simulink model "test_eb_astitsmc_comp_formation_xy_gazebo_final"  (R2023a)
settings: Solver=FixedStepAuto  StartTime=0.0  StopTime=inf  FixedStep=0.07  RelTol=1e-3
undefined symbols (not defined in the file): angular, DiscIntNeverNeededParam, linear
libraries: ros2lib x14, simulink x4, robotcorelib x4
(part 2 of 2)

== matlab function test_eb_astitsmc_comp_formation_xy_gazebo_final/Translational Control3/Flocking1/MATLAB Function ==
  data: xi input; yi input; phiAlpha output; xj input; yj input; xk input; yk input; xl input; yl input; params input

function phiAlpha  = phiAlphaFcn(xi, yi, xj, yj, xk, yk, xl, yl, params)
    
    % Flocking parameters
    epsilon = params(1); a = params(2); b = params(3); c = params(4); d = params(5); h = params(6);

    e = abs(a - b) / sqrt(4*a*b) ;

    cAlpha = sigmaNormFun(c, epsilon) ;
    dAlpha = sigmaNormFun(d, epsilon) ;

    %%
    Pi = [xi;yi] ;
    Pj = [xj;yj] ;
    Pk = [xk;yk] ;
    Pl = [xl;yl] ;

    %%
    sigmaNormj = sigmaNormFun(Pj - Pi, epsilon) ;
    nij = gradSigmaFun(Pj - Pi, epsilon) ;
    
    sigmaNormk = sigmaNormFun(Pk - Pi, epsilon) ;
    nik = gradSigmaFun(Pk - Pi, epsilon) ;

    sigmaNorml = sigmaNormFun(Pl - Pi, epsilon) ;
    nil = gradSigmaFun(Pl - Pi, epsilon) ;

    %%
    sigma1j = sigma1Fun(sigmaNormj - dAlpha + e) ;
    sigma1k = sigma1Fun(sigmaNormk - dAlpha + e) ;
    sigma1l = sigma1Fun(sigmaNorml - dAlpha + e) ;
            
    %% Position
    phiAlphaj = 0.5 * bumpFcn(sigmaNormj/cAlpha,h) * ((a+b)*sigma1j + (a-b)) ;
    phiAlphanij = phiAlphaj.* nij ;
    
    phiAlphak = 0.5 * bumpFcn(sigmaNormk/cAlpha,h) * ((a+b)*sigma1k + (a-b)) ;
    phiAlphanik = phiAlphak.* nik ;

    phiAlphal = 0.5 * bumpFcn(sigmaNorml/cAlpha,h) * ((a+b)*sigma1l + (a-b)) ;
    phiAlphanil = phiAlphal.* nil ;

    phiAlpha = phiAlphanij + phiAlphanik + phiAlphanil;

    
end

== matlab function test_eb_astitsmc_comp_formation_xy_gazebo_final/Translational Control3/Flocking1/MATLAB Function1 ==
  data: phiAlpha input; phiAlpha_int input; ui_gamma input; yaw input; Ui_pos output size=3; ui_yaw output; KP input; eyaw output size=1; eyaw1 input; eyaw2 input; eyaw4 input

function [Ui_pos, ui_yaw, eyaw]  = ctrlLaw(phiAlpha, phiAlpha_int, ui_gamma, yaw, KP, eyaw1, eyaw2, eyaw4)  %, phiBetak, bikobs, phiBetanei, bikve
    
    % Control gains and parameters
    Kx = KP(1); Ky = KP(2); Kz = KP(3);
    Kix = KP(4); Kiy = KP(5); Kiz = KP(6);
    Kyaw = KP(7); Kdyaw = KP(8);
    off = KP(9);

    eyaw = 0 - yaw(1);
    deyaw = 0 - yaw(2);


    ui_yaw = Kyaw*eyaw + Kdyaw*deyaw;
    hz_dot = ui_gamma(3,1);  %+ cBetaz * (phiBetak(3,1) + phiBetanei(3,1)) + cdBetaz * (bikobs(3,1) + bikve(3,1));

    if eyaw < off && eyaw > -off % && eyaw1 < off && eyaw1 > -off && eyaw2 < off && eyaw2 > -off && eyaw4 < off && eyaw4 > -off
        hx_dot = Kx * phiAlpha(1,1) + Kix * phiAlpha_int(1,1) + ui_gamma(1,1);  %+ cBetax * (phiBetak(1,1) + phiBetanei(1,1)) + cdBetax * (bikobs(1,1) + bikve(1,1));
        hy_dot = Ky * phiAlpha(2,1) + Kiy * phiAlpha_int(2,1) + ui_gamma(2,1);  %+ cBetay * (phiBetak(2,1) + phiBetanei(2,1)) + cdBetay * (bikobs(2,1) + bikve(2,1));
    else
        hx_dot = 0;
        hy_dot = 0;
    end
    

    Ui_pos = [hx_dot; hy_dot; hz_dot] ;
    

end

== matlab function test_eb_astitsmc_comp_formation_xy_gazebo_final/Translational Control3/Flocking1/MATLAB Function2 ==
  data: ui_prev input; xi input; yi input; zi input; ui_gamma output size=3; xr input; yr input; zr input; xr2 input; yr2 input; zr2 input; fig input; err output size=3; K_cts input; K_sw input; norm_Vex input; norm_Vey input; norm_Vez input; i_terminal input size=3; ETA input size=3; V2 input size=3; terminal output size=3; dot_ETA output size=3; dot_V2 output
function [ui_gamma, err, terminal, dot_ETA, dot_V2] = naviFeedback(ui_prev, xi, yi, zi, xr, yr, zr, xr2, yr2, zr2, fig, K_cts, K_sw, norm_Vex, norm_Vey, norm_Vez, i_terminal, ETA, V2)
    
    Kp = K_cts(1); Kpz = K_cts(2); C = K_cts(3); Cz = K_cts(4); alphaxy = K_cts(5); alphaz = K_cts(6);
    gammaxy = K_sw(1); gammaz = K_sw(2); alpha1xy = K_sw(3); alpha1z = K_sw(4); alpha2xy = K_sw(5); alpha2z = K_sw(6);

    %Sepration control
    ui_xprev = ui_prev(1); ui_yprev = ui_prev(2); ui_zprev = ui_prev(3);
    
    if fig == 1
        e_x = (xr - xi - 0.5) + (xr2 - xi - 1);
        e_y = (yr - yi - 0.5) + (yr2 - yi);
        e_z = (zr - zi + 0.1) + (zr2 - zi);
    elseif fig == 2
        e_x = (xr - xi + 0.5) + (xr2 - xi);
        e_y = (yr - yi - 0.5) + (yr2 - yi - 1);
        e_z = (zr - zi - 0.1) + (zr2 - zi);
    else
        e_x = (xr - xi + 0.5) + (xr2 - xi);
        e_y = (yr - yi - 0.5) + (yr2 - yi - 1);
        e_z = (zr - zi - 0.5) + (zr2 - zi - 0.6);
    end

    err = [e_x;e_y;e_z];

    term_1 = abs(e_x)^(alphaxy)*sign(e_x);
    term_2 = abs(e_y)^(alphaxy)*sign(e_y);
    term_3 = abs(e_z)^(alphaz)*sign(e_z);

    terminal = [term_1;term_2;term_3];

    %Manifold definitions
    Sx = e_x + C*i_terminal(1);
    Sy = e_y + C*i_terminal(2);
    Sz = e_z + Cz*i_terminal(3);

    %Disturbance estimate adaptation
    dot_eta_x = gammaxy*abs(Sx) - 0.001*ETA(1);
    dot_eta_y = gammaxy*abs(Sy) - 0.001*ETA(2);
    dot_eta_z = gammaz*abs(Sz) - 0.001*ETA(3);
    dot_ETA = [dot_eta_x;dot_eta_y;dot_eta_z];

    k1x = alpha1xy*sqrt(ETA(1));
    k1y = alpha1xy*sqrt(ETA(2));
    k1z = alpha1z*sqrt(ETA(3));

    k2x = alpha2xy*ETA(1);
    k2y = alpha2xy*ETA(2);
    k2z = alpha2z*ETA(3);

    %Switching law
    v1x = ETA(1)*tanh(Sx);
    v1y = ETA(2)*tanh(Sy);
    v1z = ETA(3)*tanh(Sz);
    
    dot_v2x = 0.001*tanh(Sx);
    dot_v2y = 0.001*tanh(Sy);
    dot_v2z = 0.0015*tanh(Sz);
    dot_V2 = [dot_v2x;dot_v2y;dot_v2z];

    % ux = 0 + v1x;
    % uy = 0 + v1y;
    % uz = 0 + v1z;

    %Final control law
    if  norm_Vex >= 0
        ux = 0 + v1x;
    else
        ux = ui_xprev;
    end

    if  norm_Vey >= 0
        uy = 0 + v1y;
    else
        uy = ui_yprev;
    end

    if  norm_Vez >= 0
        uz = 0 + v1z;
    else
        uz = ui_zprev;
    end

    ui_gamma = [ux;uy;uz];
    
end

== matlab function test_eb_astitsmc_comp_formation_xy_gazebo_final/Translational Control4/event_2 ==
  data: e_t output; X_d input; X_d2 input; X input; Kevs input; fig input
function e_t  = fcn(X_d, X_d2, X, Kevs, fig)

%Separation of desired and actual positions, velocities ans accelerations in their components
X_l = X_d(1:6); 
xr = X_l(1);    vxr = X_l(4);      
yr = X_l(2);    vyr = X_l(5);   
zr = X_l(3);    vzr = X_l(6);   

X_l2 = X_d2(1:4); 
xr2 = X_l2(1);    
yr2 = X_l2(2);    
zr2 = X_l2(3);    

X_a = X(1:3);
xi = X_a(1);     
yi = X_a(2);     
zi = X_a(3);     

%Parameters separation ans designation
c0x = Kevs(1);
c0y = Kevs(2);
c0z = Kevs(3);

%Errors definition (position and velocity)
if fig == 1
        ex = (xr - xi + 0.5) + (xr2 - xi);
        ey = (yr - yi - 0.5) + (yr2 - yi - 1);
        ez = (zr - zi - 0.1) + (zr2 - zi);
elseif fig == 2
        ex = (xr - xi + 0.5) + (xr2 - xi + 1);
        ey = (yr - yi + 0.5) + (yr2 - yi);
        ez = (zr - zi + 0.1) + (zr2 - zi);
else
        ex = (xr - xi + 0.5) + (xr2 - xi + 1);
        ey = (yr - yi + 0.5) + (yr2 - yi);
        ez = (zr - zi + 0.1) + (zr2 - zi);
end

e_x = abs(ex) - c0x;
e_y = abs(ey) - c0y;
e_z = abs(ez) - c0z;

e_t = [e_x;e_y;e_z];

== matlab function test_eb_astitsmc_comp_formation_xy_gazebo_final/Translational Control4/Flocking1/MATLAB Function ==
  data: xi input; yi input; phiAlpha output; xj input; yj input; xk input; yk input; xl input; yl input; params input

function phiAlpha  = phiAlphaFcn(xi, yi, xj, yj, xk, yk, xl, yl, params)
    
    % Flocking parameters
    epsilon = params(1); a = params(2); b = params(3); c = params(4); d = params(5); h = params(6);

    e = abs(a - b) / sqrt(4*a*b) ;

    cAlpha = sigmaNormFun(c, epsilon) ;
    dAlpha = sigmaNormFun(d, epsilon) ;

    %%
    Pi = [xi;yi] ;
    Pj = [xj;yj] ;
    Pk = [xk;yk] ;
    Pl = [xl;yl] ;

    %%
    sigmaNormj = sigmaNormFun(Pj - Pi, epsilon) ;
    nij = gradSigmaFun(Pj - Pi, epsilon) ;
    
    sigmaNormk = sigmaNormFun(Pk - Pi, epsilon) ;
    nik = gradSigmaFun(Pk - Pi, epsilon) ;

    sigmaNorml = sigmaNormFun(Pl - Pi, epsilon) ;
    nil = gradSigmaFun(Pl - Pi, epsilon) ;

    %%
    sigma1j = sigma1Fun(sigmaNormj - dAlpha + e) ;
    sigma1k = sigma1Fun(sigmaNormk - dAlpha + e) ;
    sigma1l = sigma1Fun(sigmaNorml - dAlpha + e) ;
            
    %% Position
    phiAlphaj = 0.5 * bumpFcn(sigmaNormj/cAlpha,h) * ((a+b)*sigma1j + (a-b)) ;
    phiAlphanij = phiAlphaj.* nij ;
    
    phiAlphak = 0.5 * bumpFcn(sigmaNormk/cAlpha,h) * ((a+b)*sigma1k + (a-b)) ;
    phiAlphanik = phiAlphak.* nik ;

    phiAlphal = 0.5 * bumpFcn(sigmaNorml/cAlpha,h) * ((a+b)*sigma1l + (a-b)) ;
    phiAlphanil = phiAlphal.* nil ;

    phiAlpha = phiAlphanij + phiAlphanik + phiAlphanil;

    
end

== matlab function test_eb_astitsmc_comp_formation_xy_gazebo_final/Translational Control4/Flocking1/MATLAB Function1 ==
  data: phiAlpha input; phiAlpha_int input; ui_gamma input; yaw input; Ui_pos output size=3; ui_yaw output; KP input; eyaw output size=1; eyaw1 input; eyaw2 input; eyaw3 input

function [Ui_pos, ui_yaw, eyaw]  = ctrlLaw(phiAlpha, phiAlpha_int, ui_gamma, yaw, KP, eyaw1, eyaw2, eyaw3)  %, phiBetak, bikobs, phiBetanei, bikve
    
    % Control gains and parameters
    Kx = KP(1); Ky = KP(2); Kz = KP(3);
    Kix = KP(4); Kiy = KP(5); Kiz = KP(6);
    Kyaw = KP(7); Kdyaw = KP(8);
    off = KP(9);

    eyaw = 0 - yaw(1);
    deyaw = 0 - yaw(2);


    ui_yaw = Kyaw*eyaw + Kdyaw*deyaw;
    hz_dot = ui_gamma(3,1);  %+ cBetaz * (phiBetak(3,1) + phiBetanei(3,1)) + cdBetaz * (bikobs(3,1) + bikve(3,1));

    if eyaw < off && eyaw > -off % && eyaw1 < off && eyaw1 > -off && eyaw2 < off && eyaw2 > -off && eyaw3 < off && eyaw3 > -off
        hx_dot = Kx * phiAlpha(1,1) + Kix * phiAlpha_int(1,1) + ui_gamma(1,1);  %+ cBetax * (phiBetak(1,1) + phiBetanei(1,1)) + cdBetax * (bikobs(1,1) + bikve(1,1));
        hy_dot = Ky * phiAlpha(2,1) + Kiy * phiAlpha_int(2,1) + ui_gamma(2,1);  %+ cBetay * (phiBetak(2,1) + phiBetanei(2,1)) + cdBetay * (bikobs(2,1) + bikve(2,1));
    else
        hx_dot = 0;
        hy_dot = 0;
    end
    

    Ui_pos = [hx_dot; hy_dot; hz_dot] ;
    

end

== matlab function test_eb_astitsmc_comp_formation_xy_gazebo_final/Translational Control1/Flocking1/MATLAB Function ==
  data: xi input; yi input; phiAlpha output; xj input; yj input; xk input; yk input; xl input; yl input; params input

function phiAlpha  = phiAlphaFcn(xi, yi, xj, yj, xk, yk, xl, yl, params)
    
    % Flocking parameters
    epsilon = params(1); a = params(2); b = params(3); c = params(4); d = params(5); h = params(6);

    e = abs(a - b) / sqrt(4*a*b) ;

    cAlpha = sigmaNormFun(c, epsilon) ;
    dAlpha = sigmaNormFun(d, epsilon) ;

    %%
    Pi = [xi;yi] ;
    Pj = [xj;yj] ;
    Pk = [xk;yk] ;
    Pl = [xl;yl] ;

    %%
    sigmaNormj = sigmaNormFun(Pj - Pi, epsilon) ;
    nij = gradSigmaFun(Pj - Pi, epsilon) ;
    
    sigmaNormk = sigmaNormFun(Pk - Pi, epsilon) ;
    nik = gradSigmaFun(Pk - Pi, epsilon) ;

    sigmaNorml = sigmaNormFun(Pl - Pi, epsilon) ;
    nil = gradSigmaFun(Pl - Pi, epsilon) ;

    %%
    sigma1j = sigma1Fun(sigmaNormj - dAlpha + e) ;
    sigma1k = sigma1Fun(sigmaNormk - dAlpha + e) ;
    sigma1l = sigma1Fun(sigmaNorml - dAlpha + e) ;
            
    %% Position
    phiAlphaj = 0.5 * bumpFcn(sigmaNormj/cAlpha,h) * ((a+b)*sigma1j + (a-b)) ;
    phiAlphanij = phiAlphaj.* nij ;
    
    phiAlphak = 0.5 * bumpFcn(sigmaNormk/cAlpha,h) * ((a+b)*sigma1k + (a-b)) ;
    phiAlphanik = phiAlphak.* nik ;

    phiAlphal = 0.5 * bumpFcn(sigmaNorml/cAlpha,h) * ((a+b)*sigma1l + (a-b)) ;
    phiAlphanil = phiAlphal.* nil ;

    phiAlpha = phiAlphanij + phiAlphanik + phiAlphanil;

    
end

== matlab function test_eb_astitsmc_comp_formation_xy_gazebo_final/Translational Control1/Flocking1/MATLAB Function1 ==
  data: phiAlpha input; phiAlpha_int input; ui_gamma input; yaw input; Ui_pos output size=3; ui_yaw output; KP input; eyaw output size=1; eyaw2 input; eyaw3 input; eyaw4 input

function [Ui_pos, ui_yaw, eyaw]  = ctrlLaw(phiAlpha, phiAlpha_int, ui_gamma, yaw, KP, eyaw2, eyaw3, eyaw4)  %, phiBetak, bikobs, phiBetanei, bikve
    
    % Control gains and parameters
    Kx = KP(1); Ky = KP(2); Kz = KP(3);
    Kix = KP(4); Kiy = KP(5); Kiz = KP(6);
    Kyaw = KP(7); Kdyaw = KP(8);
    off = KP(9);


    eyaw = 0 - yaw(1);
    deyaw = 0 - yaw(2);


    ui_yaw = Kyaw*eyaw + Kdyaw*deyaw;
    hz_dot = ui_gamma(3,1);  %+ cBetaz * (phiBetak(3,1) + phiBetanei(3,1)) + cdBetaz * (bikobs(3,1) + bikve(3,1));

    if eyaw < off && eyaw > -off % && eyaw2 < off && eyaw2 > -off  && eyaw3 < off && eyaw3 > -off && eyaw4 < off && eyaw4 > -off
        hx_dot = Kx * phiAlpha(1,1) + Kix * phiAlpha_int(1,1) + ui_gamma(1,1);  %+ cBetax * (phiBetak(1,1) + phiBetanei(1,1)) + cdBetax * (bikobs(1,1) + bikve(1,1));
        hy_dot = Ky * phiAlpha(2,1) + Kiy * phiAlpha_int(2,1) + ui_gamma(2,1);  %+ cBetay * (phiBetak(2,1) + phiBetanei(2,1)) + cdBetay * (bikobs(2,1) + bikve(2,1));
    else
        hx_dot = 0;
        hy_dot = 0;
    end
    

    Ui_pos = [hx_dot; hy_dot; hz_dot] ;
    

end

== matlab function test_eb_astitsmc_comp_formation_xy_gazebo_final/Translational Control1/Flocking1/MATLAB Function2 ==
  data: ui_prev input; xi input; yi input; zi input; ui_gamma output size=3; err output size=3; terminal output size=3; xr input; yr input; zr input; figure input; K_cts input; K_sw input; norm_Vex input; norm_Vey input; norm_Vez input; i_terminal input; ETA input; V2 input; dot_ETA output size=3; dot_V2 output

function [ui_gamma, err, terminal, dot_ETA, dot_V2] = naviFeedback(ui_prev, xi, yi, zi, xr, yr, zr, figure, K_cts, K_sw, norm_Vex, norm_Vey, norm_Vez, i_terminal, ETA, V2)
    
    Kp = K_cts(1); Kpz = K_cts(2); C = K_cts(3); Cz = K_cts(4); alphaxy = K_cts(5); alphaz = K_cts(6);
    gammaxy = K_sw(1); gammaz = K_sw(2); alpha1xy = K_sw(3); alpha1z = K_sw(4); alpha2xy = K_sw(5); alpha2z = K_sw(6);

    %Sepration control
    ui_xprev = ui_prev(1); ui_yprev = ui_prev(2); ui_zprev = ui_prev(3);

    if figure == 1
        e_x = xr - xi + 0.5;
        e_y = yr - yi + 0.5;
        e_z = zr - zi + 0.1;
    elseif figure == 2
        e_x = xr - xi - 0.5;
        e_y = yr - yi + 0.5;
        e_z = zr - zi - 0.1;
    else
        e_x = xr - xi - 0.5;
        e_y = yr - yi + 0.5;
        e_z = zr - zi - 0.5;
    end

    err = [e_x;e_y;e_z];

    term_1 = abs(e_x)^(alphaxy)*sign(e_x);
    term_2 = abs(e_y)^(alphaxy)*sign(e_y);
    term_3 = abs(e_z)^(alphaz)*sign(e_z);

    terminal = [term_1;term_2;term_3];

    %Manifold definitions
    Sx = e_x + C*i_terminal(1);
    Sy = e_y + C*i_terminal(2);
    Sz = e_z + Cz*i_terminal(3);

    %Disturbance estimate adaptation
    dot_eta_x = gammaxy*abs(Sx) - 0.001*ETA(1);
    dot_eta_y = gammaxy*abs(Sy) - 0.001*ETA(2);
    dot_eta_z = gammaz*abs(Sz) - 0.001*ETA(3);
    dot_ETA = [dot_eta_x;dot_eta_y;dot_eta_z];

    k1x = alpha1xy*sqrt(ETA(1));
    k1y = alpha1xy*sqrt(ETA(2));
    k1z = alpha1z*sqrt(ETA(3));

    k2x = alpha2xy*ETA(1);
    k2y = alpha2xy*ETA(2);
    k2z = alpha2z*ETA(3);

    %Switching law
    v1x = ETA(1)*tanh(Sx);
    v1y = ETA(2)*tanh(Sy);
    v1z = ETA(3)*tanh(Sz);
    
    dot_v2x = 0.001*tanh(Sx);
    dot_v2y = 0.001*tanh(Sy);
    dot_v2z = 0.0015*tanh(Sz);
    dot_V2 = [dot_v2x;dot_v2y;dot_v2z];

    % ux = 0 + v1x;
    % uy = 0 + v1y;
    % uz = 0 + v1z;

    % Final control law
    if  norm_Vex >= 0
        ux = 0 + v1x;
    else
        ux = ui_xprev;
    end

    if  norm_Vey >= 0
        uy = 0 + v1y;
    else
        uy = ui_yprev;
    end

    if  norm_Vez >= 0
        uz = 0 + v1z;
    else
        uz = ui_zprev;
    end

    ui_gamma = [ux;uy;uz];
    
end

== matlab function test_eb_astitsmc_comp_formation_xy_gazebo_final/Translational Control2/event_2 ==
  data: e_t output; X_d input; X_d2 input; X input; Kevs input; fig input
function e_t  = fcn(X_d, X_d2, X, Kevs, fig)

%Separation of desired and actual positions, velocities ans accelerations in their components
X_l = X_d(1:6); 
xr = X_l(1);    vxr = X_l(4);      
yr = X_l(2);    vyr = X_l(5);   
zr = X_l(3);    vzr = X_l(6);   

X_l2 = X_d2(1:4); 
xr2 = X_l2(1);    
yr2 = X_l2(2);    
zr2 = X_l2(3);    

X_a = X(1:3);
xi = X_a(1);     
yi = X_a(2);     
zi = X_a(3);     

%Parameters separation ans designation
c0x = Kevs(1);
c0y = Kevs(2);
c0z = Kevs(3);

%Errors definition (position and velocity)
if fig == 1
        ex = (xr - xi - 0.5) + (xr2 - xi - 1);
        ey = (yr - yi + 0.5) + (yr2 - yi + 1);
        ez = (zr - zi - 0.1) + (zr2 - zi);
elseif fig == 2
        ex = (xr - xi - 0.5) + (xr2 - xi - 1);
        ey = (yr - yi - 0.5) + (yr2 - yi - 1);
        ez = (zr - zi + 0.1) + (zr2 - zi);
else
        ex = (xr - xi - 0.5) + (xr2 - xi - 1);
        ey = (yr - yi - 0.5) + (yr2 - yi - 1);
        ez = (zr - zi + 0.1) + (zr2 - zi);
end

e_x = abs(ex) - c0x;
e_y = abs(ey) - c0y;
e_z = abs(ez) - c0z;

e_t = [e_x;e_y;e_z];

== matlab function test_eb_astitsmc_comp_formation_xy_gazebo_final/Translational Control4/event_x2 ==
  data: e_1 output; e_2 output; e1 input; e2 input; e3 input; e_3 output; i1 output; i1 input; i2 input; i3 input; i2 output; i3 output
function [e_1,e_2, e_3, i1, i2, i3]  = fcn(e1, e2, e3, i1, i2, i3)

if e1 >= 0
    e_1 = 1;
    i1 = i1+1;
else 
    e_1 = 0;
    i1 = i1;
end

if e2 >= 0
    e_2 = 1;
    i2 = i2 + 1;
else 
    e_2 = 0;
    i2 = i2;
end

if e3 >= 0
    e_3 = 1;
    i3 = i3 + 1;
else 
    e_3 = 0;
    i3 = i3;
end

== matlab function test_eb_astitsmc_comp_formation_xy_gazebo_final/Translational Control4/Flocking1/MATLAB Function2 ==
  data: ui_prev input; xi input; yi input; zi input; ui_gamma output size=3; xr input; yr input; zr input; xr2 input; yr2 input; zr2 input; fig input; err output size=3; K_cts input; K_sw input; norm_Vex input; norm_Vey input; norm_Vez input; i_terminal input size=3; ETA input size=3; V2 input size=3; terminal output size=3; dot_ETA output size=3; dot_V2 output
function [ui_gamma, err, terminal, dot_ETA, dot_V2] = naviFeedback(ui_prev, xi, yi, zi, xr, yr, zr, xr2, yr2, zr2, fig, K_cts, K_sw, norm_Vex, norm_Vey, norm_Vez, i_terminal, ETA, V2)
    
    Kp = K_cts(1); Kpz = K_cts(2); C = K_cts(3); Cz = K_cts(4); alphaxy = K_cts(5); alphaz = K_cts(6);
    gammaxy = K_sw(1); gammaz = K_sw(2); alpha1xy = K_sw(3); alpha1z = K_sw(4); alpha2xy = K_sw(5); alpha2z = K_sw(6);

    %Sepration control
    ui_xprev = ui_prev(1); ui_yprev = ui_prev(2); ui_zprev = ui_prev(3);

    if fig == 1
        e_x = (xr - xi + 0.5) + (xr2 - xi);
        e_y = (yr - yi - 0.5) + (yr2 - yi - 1);
        e_z = (zr - zi - 0.1) + (zr2 - zi);
    elseif fig == 2
        e_x = (xr - xi + 0.5) + (xr2 - xi + 1);
        e_y = (yr - yi + 0.5) + (yr2 - yi);
        e_z = (zr - zi + 0.1) + (zr2 - zi);
    else
        e_x = (xr - xi + 0.5) + (xr2 - xi + 1);
        e_y = (yr - yi + 0.5) + (yr2 - yi);
        e_z = (zr - zi + 0.1) + (zr2 - zi);
    end

    err = [e_x;e_y;e_z];

    term_1 = abs(e_x)^(alphaxy)*sign(e_x);
    term_2 = abs(e_y)^(alphaxy)*sign(e_y);
    term_3 = abs(e_z)^(alphaz)*sign(e_z);

    terminal = [term_1;term_2;term_3];

    %Manifold definitions
    Sx = e_x + C*i_terminal(1);
    Sy = e_y + C*i_terminal(2);
    Sz = e_z + Cz*i_terminal(3);

    %Disturbance estimate adaptation
    dot_eta_x = gammaxy*abs(Sx) - 0.001*ETA(1);
    dot_eta_y = gammaxy*abs(Sy) - 0.001*ETA(2);
    dot_eta_z = gammaz*abs(Sz) - 0.001*ETA(3);
    dot_ETA = [dot_eta_x;dot_eta_y;dot_eta_z];

    k1x = alpha1xy*sqrt(ETA(1));
    k1y = alpha1xy*sqrt(ETA(2));
    k1z = alpha1z*sqrt(ETA(3));

    k2x = alpha2xy*ETA(1);
    k2y = alpha2xy*ETA(2);
    k2z = alpha2z*ETA(3);

    %Switching law
    v1x = ETA(1)*tanh(Sx);
    v1y = ETA(2)*tanh(Sy);
    v1z = ETA(3)*tanh(Sz);
    
    dot_v2x = 0.001*tanh(Sx);
    dot_v2y = 0.001*tanh(Sy);
    dot_v2z = 0.0015*tanh(Sz);
    dot_V2 = [dot_v2x;dot_v2y;dot_v2z];

    % ux = 0 + v1x;
    % uy = 0 + v1y;
    % uz = 0 + v1z;

    % Final control law
    if  norm_Vex >= 0
        ux = 0 + v1x;
    else
        ux = ui_xprev;
    end

    if  norm_Vey >= 0
        uy = 0 + v1y;
    else
        uy = ui_yprev;
    end

    if  norm_Vez >= 0
        uz = 0 + v1z;
    else
        uz = ui_zprev;
    end

    ui_gamma = [ux;uy;uz];
    
end

== matlab function test_eb_astitsmc_comp_formation_xy_gazebo_final/Translational Control1/event_2 ==
  data: e_t output; X_d input; X input; Kevs input; figure input
function e_t  = fcn(X_d, X, Kevs, figure)

%Separation of desired and actual positions, velocities ans accelerations in their components
X_l = X_d(1:6); 
xr = X_l(1);    vxr = X_l(4);      
yr = X_l(2);    vyr = X_l(5);   
zr = X_l(3);    vzr = X_l(6);   

X_a = X(1:3);
xi = X_a(1);     
yi = X_a(2);     
zi = X_a(3);     

%Parameters separation ans designation
c0x = Kevs(1);
c0y = Kevs(2);
c0z = Kevs(3);

%Errors definition (position and velocity)
if figure == 1
        ex = xr - xi + 0.5;
        ey = yr - yi + 0.5;
        ez = zr - zi + 0.1;
elseif figure == 2
        ex = xr - xi - 0.5;
        ey = yr - yi + 0.5;
        ez = zr - zi - 0.1;
else
        ex = xr - xi - 0.5;
        ey = yr - yi + 0.5;
        ez = zr - zi - 0.5;
end

e_x = abs(ex) - c0x;
e_y = abs(ey) - c0y;
e_z = abs(ez) - c0z;

e_t = [e_x;e_y;e_z];

== matlab function test_eb_astitsmc_comp_formation_xy_gazebo_final/Translational Control1/event_x2 ==
  data: e_1 output; e_2 output; e1 input; e2 input; e3 input; e_3 output; i1 output; i1 input; i2 input; i3 input; i2 output; i3 output
function [e_1,e_2, e_3, i1, i2, i3]  = fcn(e1, e2, e3, i1, i2, i3)

if e1 >= 0
    e_1 = 1;
    i1 = i1+1;
else 
    e_1 = 0;
    i1 = i1;
end

if e2 >= 0
    e_2 = 1;
    i2 = i2 + 1;
else 
    e_2 = 0;
    i2 = i2;
end

if e3 >= 0
    e_3 = 1;
    i3 = i3 + 1;
else 
    e_3 = 0;
    i3 = i3;
end

== matlab function test_eb_astitsmc_comp_formation_xy_gazebo_final/Subsystem/MATLAB Function6 ==
  data: X1 input; X2 input; X3 input; d_meas input; xyz output
function xyz = fcn(X1, X2, X3, d_meas)

%% Extract data from vectors
states1 = X1(1:3);
x1 = states1(1);
y1 = states1(2);
z1 = states1(3);

states2 = X2(1:3);
x2 = states2(1);
y2 = states2(2);
z2 = states2(3);

states3 = X3(1:3);
x3 = states3(1);
y3 = states3(2);
z3 = states3(3);

r1 = d_meas(1);
r2 = d_meas(2);
r3 = d_meas(3);

xyz = multi_fun(x1, y1, r1, x2, y2, r2, x3, y3, r3);

== matlab function test_eb_astitsmc_comp_formation_xy_gazebo_final/Translational Control2/event_x2 ==
  data: e1 input; e2 input; e3 input; i1 output; i1 input; i2 input; i3 input; i2 output; i3 output
function [i1, i2, i3]  = fcn(e1, e2, e3, i1, i2, i3)

if e1 >= 0
    e_1 = 1;
    i1 = i1+1;
else 
    e_1 = 0;
    i1 = i1;
end

if e2 >= 0
    e_2 = 1;
    i2 = i2 + 1;
else 
    e_2 = 0;
    i2 = i2;
end

if e3 >= 0
    e_3 = 1;
    i3 = i3 + 1;
else 
    e_3 = 0;
    i3 = i3;
end

== matlab function test_eb_astitsmc_comp_formation_xy_gazebo_final/Translational Control3/event_x2 ==
  data: e1 input; e2 input; e3 input; i1 output; i1 input; i2 input; i3 input; i2 output; i3 output
function [i1, i2, i3]  = fcn(e1, e2, e3, i1, i2, i3)

if e1 >= 0
    e_1 = 1;
    i1 = i1+1;
else 
    e_1 = 0;
    i1 = i1;
end

if e2 >= 0
    e_2 = 1;
    i2 = i2 + 1;
else 
    e_2 = 0;
    i2 = i2;
end

if e3 >= 0
    e_3 = 1;
    i3 = i3 + 1;
else 
    e_3 = 0;
    i3 = i3;
end

== matlab function test_eb_astitsmc_comp_formation_xy_gazebo_final/continuous ==
  data: i output; t input; tp input; tp output; i input
function [i,tp] = fcn(t,tp,i)


%u = 0.1*cos(1.5*t) + 0.05*sin(t);         % x-component of vector field
%v = 0.1*sin(3*t) - 0.06*sin(0.5*t);      % y-component of vector field
if t > tp
    i = i + 1;
else 
    i = i;
end

== matlab function test_eb_astitsmc_comp_formation_xy_gazebo_final/MATLAB Function1 ==
  data: sec input; gaz_time output; nanosec input
function gaz_time = fcn(sec, nanosec)

nanosec1 = double(nanosec)/1000000000; %*10^(-9);

sec1 = double(sec);

gaz_time = sec1 + nanosec1;
